simulink model "subsampling4"  (R2021a)
settings: Solver=VariableStepAuto  StartTime=0.0  StopTime=0.1  MaxStep=1/10e6  RelTol=1e-3
undefined symbols (not defined in the file or in its folder): a, b
libraries: dspsigops x3, simulink x1, dspstat3 x1
settings Model: Creator=josef  LastModifiedBy=josef
settings SolverCC: AlgebraicLoopSolver=TrustRegion
settings DebuggingCC: SFMachineParentedDataDiag=warning

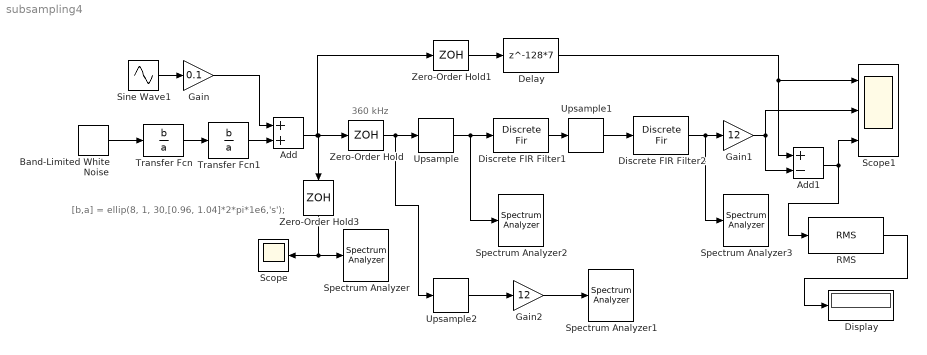
== system subsampling4 ==
  note: [b,a] = ellip(8, 1, 30,[0.96, 1.04]*2*pi*1e6,'s');
  note: 360 kHz
  Add : Sum
  Add1 : Sum  Inputs=+-
  Band-Limited White Noise : simulink/Sources/Band-Limited White Noise  Cov=1/3e6  Ts=1/3e6  seed=[23341]
  Delay : Delay  DelayLength=128*7
  Discrete FIR Filter1 : DiscreteFir  Coefficients=fir1(256,[0.180,0.350]*2/0.72)
  Discrete FIR Filter2 : DiscreteFir  Coefficients=fir1(256,[0.9,1.09]*2/4.32)
  Display : Display
  Gain : Gain  Gain=0.1
  Gain1 : Gain  Gain=12
  Gain2 : Gain  Gain=12
  RMS : dspstat3/RMS  run=on  directionMode=Each column  dimension=1  reset_popup=None
  Scope : Scope
  Scope1 : Scope  NumInputPorts=3
  Sine Wave1 : Sin  Frequency=2*pi*0.99e6  SampleTime=0
  Spectrum Analyzer{,1..3} (4 alike) : SpectrumAnalyzer
  Transfer Fcn : TransferFcn  Numerator=b  Denominator=a
  Transfer Fcn1 : TransferFcn  Numerator=b  Denominator=a
  Upsample : dspsigops/Upsample  N=2  phase=0  RateOptions=Allow multirate processing  ic=0  mode=Unused parameter value
  Upsample1 : dspsigops/Upsample  N=6  phase=0  RateOptions=Allow multirate processing  ic=0  mode=Unused parameter value
  Upsample2 : dspsigops/Upsample  N=12  phase=0  RateOptions=Allow multirate processing  ic=0  mode=Unused parameter value
  Zero-Order Hold : ZeroOrderHold  SampleTime=1/360e3
  Zero-Order Hold1 : ZeroOrderHold  SampleTime=1/4.32e6
  Zero-Order Hold3 : ZeroOrderHold  SampleTime=1/3e6
  wires:
  Zero-Order Hold1/1 -> Delay/1
  Delay/1 -> Add1/1, Scope1/1
  Band-Limited White Noise/1 -> Transfer Fcn/1
  Sine Wave1/1 -> Gain/1
  Add/1 -> Zero-Order Hold3/1, Zero-Order Hold/1, Zero-Order Hold1/1
  Zero-Order Hold3/1 -> Spectrum Analyzer/1, Scope/1
  Gain/1 -> Add/1
  Transfer Fcn/1 -> Transfer Fcn1/1
  Discrete FIR Filter1/1 -> Upsample1/1
  Gain1/1 -> Scope1/2, Add1/2
  Upsample1/1 -> Discrete FIR Filter2/1
  Discrete FIR Filter2/1 -> Spectrum Analyzer3/1, Gain1/1
  Zero-Order Hold/1 -> Upsample2/1, Upsample/1
  RMS/1 -> Display/1
  Upsample/1 -> Discrete FIR Filter1/1, Spectrum Analyzer2/1
  Transfer Fcn1/1 -> Add/2
  Upsample2/1 -> Gain2/1
  Gain2/1 -> Spectrum Analyzer1/1
  Add1/1 -> Scope1/3, RMS/1
